simulink model "incremental_rst_sim"  (R2023a)
settings: Solver=VariableStepAuto  StartTime=0.0  StopTime=5  RelTol=1e-3
undefined symbols (not defined in the file): delay, K, r, s, tau, ts
settings Model: Creator=ACER  LastModifiedBy=ACER

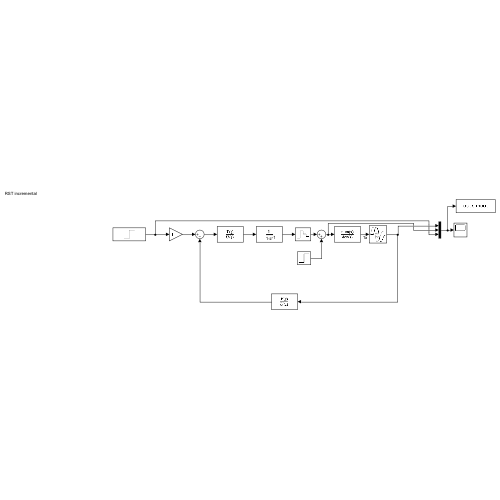
[thumbnail: Simulink's stored preview of the top-level diagram]
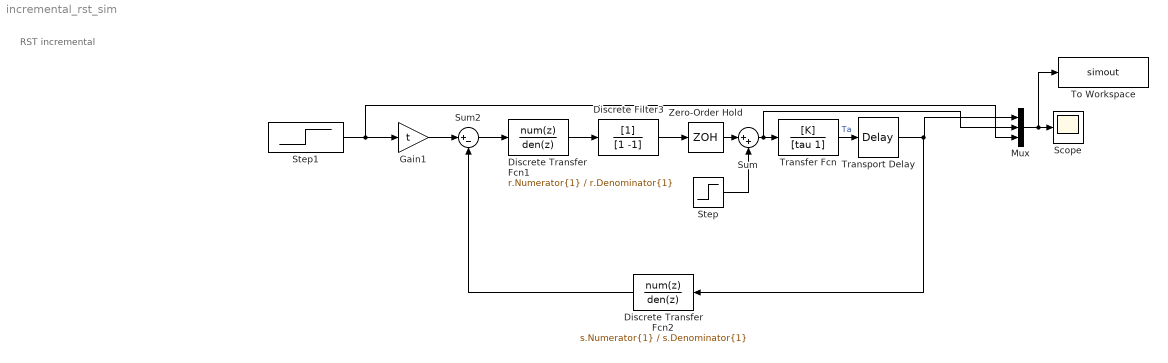
== system incremental_rst_sim ==
  note: RST incremental
  Discrete Transfer Fcn1 : DiscreteTransferFcn  Numerator=r.Numerator{1}  Denominator=r.Denominator{1}  SampleTime=ts
  Discrete Transfer Fcn2 : DiscreteTransferFcn  Numerator=s.Numerator{1}  Denominator=s.Denominator{1}  SampleTime=ts
  Discrete Filter3 : DiscreteFilter  Denominator=[1 -1]
  Gain1 : Gain  Gain=t
  Mux : Mux  Inputs=3
  Scope : Scope
  Step : Step  Time=3  After=10  SampleTime=0
  Step1 : Step  Time=0  After=40  SampleTime=0
  Sum : Sum  Inputs=|++
  Sum2 : Sum  Inputs=|+-
  To Workspace : ToWorkspace  VariableName=simout  SaveFormat=Timeseries  SampleTime=-1
  Transfer Fcn : TransferFcn  Numerator=[K]  Denominator=[tau 1]
  Transport Delay : TransportDelay  DelayTime=delay
  Zero-Order Hold : ZeroOrderHold  SampleTime=ts
  wires:
  Step1/1 -> Mux/3, Gain1/1
  Sum2/1 -> Discrete Transfer Fcn1/1
  Discrete Transfer Fcn2/1 -> Sum2/2
  Discrete Transfer Fcn1/1 -> Discrete Filter3/1
  Gain1/1 -> Sum2/1
  Discrete Filter3/1 -> Zero-Order Hold/1
  Transport Delay/1 -> Mux/1, Discrete Transfer Fcn2/1
  Mux/1 -> To Workspace/1, Scope/1
  Transfer Fcn/1 -> Transport Delay/1  "Ta"
  Zero-Order Hold/1 -> Sum/1
  Sum/1 -> Mux/2, Transfer Fcn/1
  Step/1 -> Sum/2
